simulink model "pendilum"  (R2026a)
settings: Solver=ode4  StopTime=5  FixedStep=0.01
values from neighbouring files (symbols this model uses):
  A = M + m    (= 2)    [run_pendilum.m]
  b_0 = 0.1    [run_pendilum.m]
  b_z = 0    [run_pendilum.m]
  C = J + m * l^2    (= 0.045)    [run_pendilum.m]
  F_max = 10    [run_pendilum.m]
  g = 9.81    [run_pendilum.m]
  Kd = 2    [run_pendilum.m]
  Kp = 30    [run_pendilum.m]
  Kv = 0.15    [run_pendilum.m]
  Kz = 0.05    [run_pendilum.m]
  l = 0.15    [run_pendilum.m]
  m = 1.5    [run_pendilum.m]
  phi_0 = 5*pi/180    (= 0.0872664625997)    [run_pendilum.m]
  Pos_limit = 5*pi/180    (= 0.0872664625997)    [run_pendilum.m]
  z_ref = 0    [run_pendilum.m]
libraries: slpidlib x1
settings Model: Creator=vb  LastModifiedBy=vb

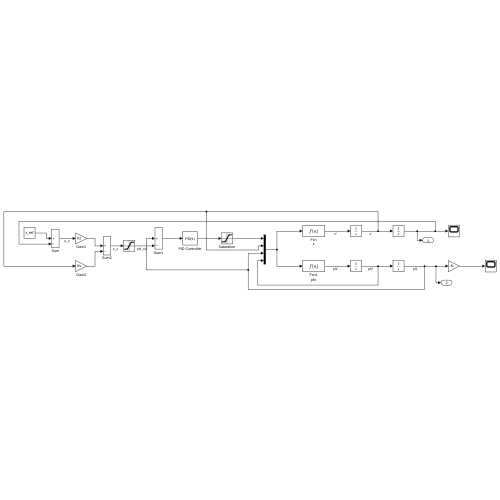
[thumbnail: Simulink's stored preview of the top-level diagram]
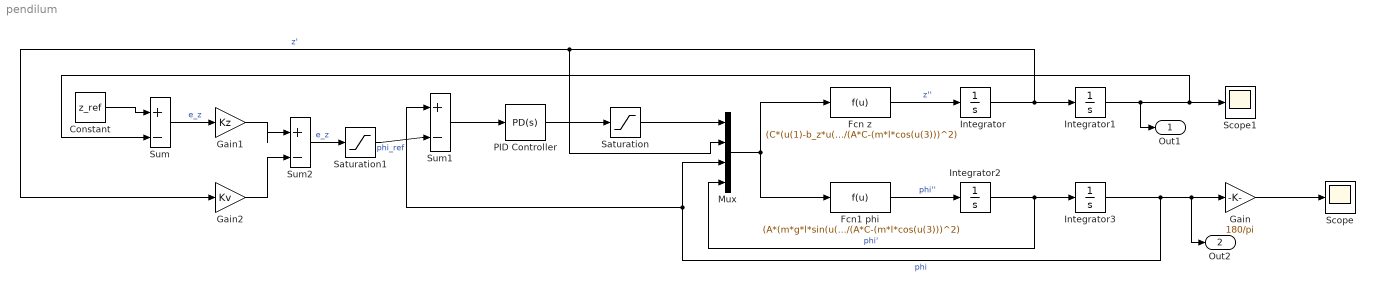
== system pendilum ==
  Constant : Constant  Value=z_ref
  Fcn z : Fcn  Expr=(C*(u(1)-b_z*u(2)+m*l*u(4)^2*sin(u(3)))-(m*l*cos(u(3)))*(m*g*l*sin(u(3))-b_0*u(4)))/(A*C-(m*l*cos(u(3)))^2)
  Fcn1 phi : Fcn  Expr=(A*(m*g*l*sin(u(3))-b_0*u(4))-(m*l*cos(u(3)))*(u(1)-b_z*u(2)+m*l*u(4)^2*sin(u(3))))/(A*C-(m*l*cos(u(3)))^2)
  Gain : Gain  Gain=180/pi
  Gain1 : Gain  Gain=Kz
  Gain2 : Gain  Gain=Kv
  Integrator : Integrator
  Integrator1 : Integrator
  Integrator2 : Integrator
  Integrator3 : Integrator  InitialCondition=phi_0
  Mux : Mux
  PID Controller : slpidlib/PID Controller  Controller=PD  Form=Parallel  TimeDomain=Continuous-time  UseExternalTs=off  SampleTime=-1  IntegratorMethod=Forward Euler  FilterMethod=Forward Euler  ControllerParametersSource=internal  P=Kp  I=1  UseKiTs=off  D=Kd  UseExternalDerivativeSource=off  N=100  UseFilter=on  TunerSelectOption=Transfer Function Based (PID Tuner App)  InitialConditionSource=internal  InitialConditionForIntegrator=0  InitialConditionForFilter=0  DifferentiatorICPrevScaledInput=0  ExternalReset=none  TrackingMode=off  Kt=1  LimitOutput=off  SatLimitsSource=internal  UpperSaturationLimit=inf  LowerSaturationLimit=-inf  LinearizeAsGain=on  AntiWindupMode=none  Kb=1  LimitIntegrator=off  UpperIntegratorSaturationLimit=inf  LowerIntegratorSaturationLimit=-inf  POutMin=[]  POutMax=[]  IOutMin=[]  IOutMax=[]  DOutMin=[]  DOutMax=[]  NOutMin=[]  NOutMax=[]  SumOutMin=[]  SumOutMax=[]  SaturationOutMin=[]  SaturationOutMax=[]  PParamMin=[]  PParamMax=[]  IParamMin=[]  IParamMax=[]  DParamMin=[]  DParamMax=[]  NParamMin=[]  NParamMax=[]  KbParamMin=[]  KbParamMax=[]  KtParamMin=[]  KtParamMax=[]  KbOutMin=[]  KbOutMax=[]  KtOutMin=[]  KtOutMax=[]  IntegratorOutMin=[]  IntegratorOutMax=[]  FilterOutMin=[]  FilterOutMax=[]  SumI1OutMin=[]  SumI1OutMax=[]  SumI2OutMin=[]  SumI2OutMax=[]  SumI3OutMin=[]  SumI3OutMax=[]  SumI4OutMin=[]  SumI4OutMax=[]  SumDOutMin=[]  SumDOutMax=[]  DifferentiatorOutMin=[]  DifferentiatorOutMax=[]  FilterDiffOutCoefMin=[]  FilterDiffOutCoefMax=[]  ReciprocalOutMin=[]  ReciprocalOutMax=[]  SumDenOutMin=[]  SumDenOutMax=[]  SumNumOutMin=[]  SumNumOutMax=[]  DivideOutMin=[]  DivideOutMax=[]  UdiffTsProdOutMin=[]  UdiffTsProdOutMax=[]  NTsProdOutMin=[]  NTsProdOutMax=[]  UintegralTsProdOutMin=[]  UintegralTsProdOutMax=[]  UngainTsProdOutMin=[]  UngainTsProdOutMax=[]  ClampingZeroOutDataTypeStr=Inherit: Inherit via back propagation  ClampingZeroOutMin=[]  ClampingZeroOutMax=[]  FilterDenConstantOutDataTypeStr=Inherit: Inherit via back propagation  FilterDenConstantOutMin=[]  FilterDenConstantOutMax=[]  PCopyOutDataTypeStr=Inherit: Inherit via back propagation  PCopyOutMin=[]  PCopyOutMax=[]  NCopyOutDataTypeStr=Inherit: Inherit via back propagation  NCopyOutMin=[]  NCopyOutMax=[]  IntegratorContinuousStateAttributes=''  IntegratorStateMustResolveToSignalObject=off  IntegratorRTWStateStorageClass=Auto  FilterContinuousStateAttributes=''  FilterStateMustResolveToSignalObject=off  FilterRTWStateStorageClass=Auto  ParallelPVariant=InternalParameters  IdealPVariant=Disabled  IVariant=Disabled  DVariant=InternalParameters  IntegratorVariant=Disabled  SatVariant=Disabled  AWVariant=Disabled  PCopyVariant=Disabled  TRVariant=Disabled  FdbkBlocksVariant=Forward  IdealPFdbkVariant=Disabled  SatFdbkVariant=Disabled  DerivativeFilterVariant=ContFilter  NVariant=InternalParameters  NCopyVariant=Disabled  FilterICVariant=InternalICsFilter  IntegratorICVariant=Disabled  ExternalResetVariant=Disabled  TRSumVariant=Passthrough  SumFdbkVariant=Disabled  SumVariant=Sum_PD  TsampFilterVariant=InternalTs  TsampNgainVariant=Passthrough  TsampIntegralVariant=Disabled_SignalSpec  ExternalSaturationOutDataTypeStr=Inherit: Same as second input  DerivativeSourceVariant=ErrorSignal  PreIntVariant=InternalPreInt
  Saturation : Saturate  UpperLimit=F_max  LowerLimit=-F_max
  Saturation1 : Saturate  UpperLimit=Pos_limit  LowerLimit=-Pos_limit
  Scope : Scope
      settings: ActiveDisplayYMinimum=-15.150791875894797  ActiveDisplayYMaximum=66.327744399096275
  Scope1 : Scope
      settings: ActiveDisplayYMinimum=-1.5015930230579662  ActiveDisplayYMaximum=2.0054566218010748
  Sum : Sum  Inputs=|+-
  Sum1 : Sum  Inputs=|+-
  Sum2 : Sum  Inputs=|+-
  Out1 : Outport
  Out2 : Outport  Port=2
  wires:
  Mux/1 -> Fcn z/1, Fcn1 phi/1
  Fcn z/1 -> Integrator/1  "z''"
  Integrator/1 -> Gain2/1, Mux/2, Integrator1/1  "z'"
  Fcn1 phi/1 -> Integrator2/1  "phi''"
  Integrator2/1 -> Mux/4, Integrator3/1  "phi'"
  Integrator3/1 -> Out2/1, Gain/1, Sum1/1, Mux/3  "phi"
  Integrator1/1 -> Out1/1, Sum/2, Scope1/1
  Gain/1 -> Scope/1
  PID Controller/1 -> Saturation/1
  Constant/1 -> Sum/1
  Sum/1 -> Gain1/1  "e_z"
  Sum1/1 -> PID Controller/1
  Saturation1/1 -> Sum1/2  "phi_ref"
  Saturation/1 -> Mux/1
  Sum2/1 -> Saturation1/1  "e_z"
  Gain1/1 -> Sum2/1
  Gain2/1 -> Sum2/2
